simulink model "currentGenerator"  (R2016a)
settings: Solver=VariableStepAuto  StartTime=0.0  StopTime=10.0  RelTol=1e-3
settings Model: Creator=enes_  LastModifiedBy=enes_

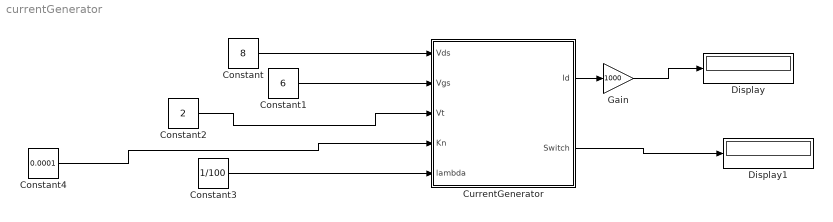
== system currentGenerator ==
  Constant : Constant  Value=8
  Constant1 : Constant  Value=6
  Constant2 : Constant  Value=2
  Constant3 : Constant  Value=1/100
  Constant4 : Constant  Value=0.0001
  CurrentGenerator : MATLAB Function  TreatAsAtomicUnit=on
  Display : Display
  Display1 : Display
  Gain : Gain  Gain=1000
  wires:
  Constant/1 -> CurrentGenerator/1(Vds)
  Constant1/1 -> CurrentGenerator/2(Vgs)
  Constant2/1 -> CurrentGenerator/3(Vt)
  Constant3/1 -> CurrentGenerator/5(lambda)
  Constant4/1 -> CurrentGenerator/4(Kn)
  CurrentGenerator/2(Switch) -> Display1/1
  CurrentGenerator/1(Id) -> Gain/1
  Gain/1 -> Display/1

== matlab function currentGenerator/CurrentGenerator ==
  data: Vds input; Id output; Vgs input; Vt input; Kn input; lambda input; Switch output
function [Id,Switch] = fcn(Vds,Vgs,Vt,Kn,lambda)
%#codegen
% Vds: Drain-to-source voltage in V
% Vgs: Gate-to-source voltage in V
% Vt: Threshold Voltage in V
% Kn: Devices parameter in A/V^2
% Lambda: Early voltage in V^-1

% Id: Drain-to-Source Current
% Switch : determines the on-off state of switch
Current=0;
SwitchStat=0;
GSVt= Vgs-Vt; % it determines transistor on or off

OnStat=Vds-Vgs+Vt; % it determines transistor is sat or linear

if GSVt>0
    
    if OnStat>0
        % SaturationRegion
       Current = 0.5*Kn*(GSVt^2)*(1+lambda*Vds);
       SwitchStat= 0;
    else
        % Triode region
        Current=Kn*((GSVt*Vds)-(0.5*Vds*Vds))*(1+lambda*Vds);
        SwitchStat=1;
        
    end
    
    
    
    
else
    % cut-off region
    Current=0;
    SwitchStat=0;
    
end

Id=Current;
Switch=SwitchStat;
